simulink model "linear_validation"  (R2017b)
settings: Solver=VariableStepAuto  StartTime=0.0  StopTime=10.0  RelTol=1e-3
undefined symbols (not defined in the file): system
settings Model: Creator=Twan  LastModifiedBy=Twan

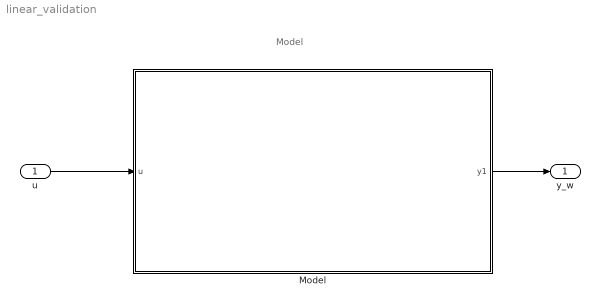
== system linear_validation ==
  note: Model
  u : Inport
  Model : Subsystem
  "y_w " : Outport
  wires:
  Model/1(y1) -> "y_w "/1
  u/1 -> Model/1(u)

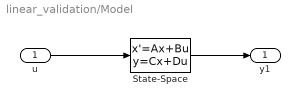
== system linear_validation/Model ==
  u : Inport
  State-Space : StateSpace  A=system.ss.lin.A  B=system.ss.lin.B  C=system.ss.lin.C  D=system.ss.lin.D  InitialCondition=[1]
  y1 : Outport
  wires:
  u/1 -> State-Space/1
  State-Space/1 -> y1/1
